simulink library "thermochemical"  (R2017b)
settings: Solver=VariableStepAuto  StartTime=0.0  StopTime=10.0  RelTol=1e-3
values from neighbouring files (symbols this model uses):
  c = conversion_factors()    [blk_clausius_clapeyron.m]    (also in blk_clausius_clapeyron_no_popup.m; blk_cold_room_closed_dry_air.m; blk_reactor_BaCl2_NH3_no_walls.m; blk_reactor_BaCl2_NH3_no_walls_state_space.m)
  cp = metal.cp    [blk_wall_simple.m]    (also in get_metal_properties.m = 390)
  fluid = get_param(blk,'fluid')    [blk_thermodynamic_properties_nonsaturated.m]    (also in blk_thermodynamic_properties_nonsaturated_interpreted.m; blk_thermodynamic_properties_saturated.m; blk_thermodynamic_properties_saturated_interpreted.m; blk_thermodynamic_properties_saturated_mix.m)
  gas = get_material_properties(x.gasName)    [blk_reactor_BaCl2_NH3_cylindrical_no_walls_fun1.m]
  h = get_param(gcb,'ObjectParameters')    [get_param_eval.m]
  rho = metal.rho    [blk_wall_simple.m]    (also in get_metal_properties.m = 8940)
  s = solve(eq,dx,'ReturnConditions',true)    [LMTD_inv.m]    (also in blk_wall_simple.m = get_param_eval(blk,'s'))
  u_gas_at_T_ref = -R * T_ref    [blk_reactor_BaCl2_NH3_no_walls.m]    (also in blk_reactor_BaCl2_NH3_no_walls_state_space.m)
undefined symbols (not defined in the file or in its folder): b_motor, BaCl2, beta, CoolProp, cP_binder, cP_gas, cP_s0, cv, dh_r_0, ENG, heat_exchanger_epsilonNTU_inv_simulink, heat_exchanger_epsilonNTU_simulink, J_motor, K_cin, kappa, Km_motor, La_motor, lookup2D_BreakPoint2, M_binder, N_binder, N_gas_free_volume_init, N_salt, NH3, nh3_v3, nu, P, phase, PID_D_motor, PID_I_motor, PID_P_motor, Ra_motor, Reactor_phase, T, T1, T2, T_init, Tr_init, Tr_ref, U_binder_at_Tr_ref, U_salt_at_X0_Tr_ref, Ur_init, V_void, Valve_regime, Vmax_motor, w_init_motor, X_init
libraries: thermochemical x247, simulink x54, dspsigops x3
(part 3 of 12)

== system thermochemical/Control volumes/Two-phase saturated fluid control volume (with wall, simple) (without algebraic loop) ==
  In2 : Inport
  In5 : Inport  Port=2
  In6 : Inport  Port=3
  In7 : Inport  Port=4
  In1 : Inport  Port=5
  In3 : Inport  Port=6
  In4 : Inport  Port=7
  In8 : Inport  Port=8
  Gain : Gain  Gain=-1
  Subsystem2 : Subsystem
  Two-phase saturated fluid control volume (without walls) (without algebraic loop) : thermochemical/Control volumes/Two-phase saturated fluid control volume (without walls) (without algebraic loop)  N_init=100  T_init=300  fluid=fluid  V=0.01
      settings: SourceProductName=@ Thermochemical
  "Wall, simple, h as inputs" : thermochemical/Walls/Wall, simple, h as inputs  material=Aluminum 1100  cp=905.9  rho=2658  s=1  e_mm=1  mass=2.658  Twall_init=300
      settings: SourceProductName=@ Thermochemical
  Out6 : Outport
  Out4 : Outport  Port=2
  Out11 : Outport  Port=3
  Out7 : Outport  Port=4
  Out5 : Outport  Port=5
  Out12 : Outport  Port=6
  Out13 : Outport  Port=7
  Out8 : Outport  Port=8
  Out1 : Outport  Port=9
  Out10 : Outport  Port=10
  wires:
  In1/1 -> Two-phase saturated fluid control volume (without walls) (without algebraic loop)/5  "dn/dt liq,out (mol/sec) (must be >= 0 !)"
  Gain/1 -> Two-phase saturated fluid control volume (without walls) (without algebraic loop)/1
  In2/1 -> "Wall, simple, h as inputs"/1  "T outer (K)"
  "Wall, simple, h as inputs"/3 -> Out13/1  "q wall → outer (W)"
  In6/1 -> Two-phase saturated fluid control volume (without walls) (without algebraic loop)/3  "dn/dt in (mol/sec) (must be >= 0 !)"
  In5/1 -> Two-phase saturated fluid control volume (without walls) (without algebraic loop)/2  "h in (J/mol)"
  Two-phase saturated fluid control volume (without walls) (without algebraic loop)/3 -> Out5/1, Subsystem2/3(In1)  "liquid volumetric fraction (0..1)"
  Two-phase saturated fluid control volume (without walls) (without algebraic loop)/4 -> Out7/1  "vapor quality (0..1)"
  Two-phase saturated fluid control volume (without walls) (without algebraic loop)/5 -> Out8/1  "h vap (sat) (J/mol)"
  In7/1 -> Two-phase saturated fluid control volume (without walls) (without algebraic loop)/4  "dn/dt vap,out (mol/sec) (must be >= 0 !)"
  Two-phase saturated fluid control volume (without walls) (without algebraic loop)/6 -> Out10/1  "h liq+vap (sat) (J/mol)"
  Two-phase saturated fluid control volume (without walls) (without algebraic loop)/2 -> Out6/1  "P sat (bar)"
  Two-phase saturated fluid control volume (without walls) (without algebraic loop)/1 -> Out4/1, "Wall, simple, h as inputs"/3  "T sat (K)"
  Two-phase saturated fluid control volume (without walls) (without algebraic loop)/7 -> Out1/1  "h liq (sat) (J/mol)"
  "Wall, simple, h as inputs"/1 -> Out11/1  "T wall (K)"
  "Wall, simple, h as inputs"/2 -> Out12/1, Gain/1  "q inner → wall (W)"
  Subsystem2/1(Out1) -> "Wall, simple, h as inputs"/4
  In8/1 -> Subsystem2/2(In3)  "h inner,vap (W/m²/K)"
  In4/1 -> Subsystem2/1(In2)  "h inner,liq (W/m²/K)"
  In3/1 -> "Wall, simple, h as inputs"/2  "h outer (W/m²/K)"

== system thermochemical/Control volumes/Two-phase saturated fluid control volume (with wall, tube with//without fins) ==
  In2 : Inport
  In5 : Inport  Port=2
  In6 : Inport  Port=3
  In7 : Inport  Port=4
  In1 : Inport  Port=5
  In3 : Inport  Port=6
  In4 : Inport  Port=7
  In8 : Inport  Port=8
  Display : Display
  Gain : Gain  Gain=-1
  Subsystem2 : Subsystem
  Two-phase saturated fluid control volume (without walls) : thermochemical/Control volumes/Two-phase saturated fluid control volume (without walls)  N_init=100  T_init=300  fluid=fluid  V=0.01
      settings: SourceProductName=@ Thermochemical
  "Wall, tube with/without fins" : thermochemical/Walls/Wall, tube with//without fins  L_m=1  OD_mm=10  e_mm=1  material_tube=Aluminum 1100  cp_tube=905.9  rho_tube=2658  height_fin_mm=0  thickness_fin_mm=0  pitch_fin_mm=0  material_fin=Aluminum 1100  cp_fin=905.9  rho_fin=2658  lambda_fin=211.8  Tinit=300  mass_tube=0.039664  mass_fin=0  mass_total=0.039664  s_inner=0.028274  s_outer=0.031416
      settings: SourceProductName=@ Thermochemical
  Out6 : Outport
  Out4 : Outport  Port=2
  Out11 : Outport  Port=3
  Out7 : Outport  Port=4
  Out5 : Outport  Port=5
  Out12 : Outport  Port=6
  Out13 : Outport  Port=7
  Out8 : Outport  Port=8
  Out1 : Outport  Port=9
  Out10 : Outport  Port=10
  wires:
  Gain/1 -> Two-phase saturated fluid control volume (without walls)/1
  In2/1 -> "Wall, tube with/without fins"/1  "T outer (K)"
  "Wall, tube with/without fins"/3 -> Out13/1  "q wall → outer (W)"
  Two-phase saturated fluid control volume (without walls)/3 -> Out5/1, Subsystem2/3(In1)  "liquid volumetric fraction (0..1)"
  Two-phase saturated fluid control volume (without walls)/4 -> Out7/1  "vapor quality (0..1)"
  Two-phase saturated fluid control volume (without walls)/5 -> Out8/1  "h vap (sat) (J/mol)"
  Two-phase saturated fluid control volume (without walls)/6 -> Out10/1  "h liq+vap (sat) (J/mol)"
  Two-phase saturated fluid control volume (without walls)/2 -> Out6/1  "P sat (bar)"
  Two-phase saturated fluid control volume (without walls)/1 -> "Wall, tube with/without fins"/3, Out4/1  "T sat (K)"
  Two-phase saturated fluid control volume (without walls)/7 -> Out1/1  "h liq (sat) (J/mol)"
  "Wall, tube with/without fins"/1 -> Out11/1  "T wall (K)"
  "Wall, tube with/without fins"/2 -> Gain/1, Out12/1  "q inner → wall (W)"
  Subsystem2/1(Out1) -> "Wall, tube with/without fins"/4
  "Wall, tube with/without fins"/4 -> Display/1
  In6/1 -> Two-phase saturated fluid control volume (without walls)/3  "dn/dt in (mol/sec) (must be >= 0 !)"
  In7/1 -> Two-phase saturated fluid control volume (without walls)/4  "dn/dt vap,out (mol/sec) (must be >= 0 !)"
  In5/1 -> Two-phase saturated fluid control volume (without walls)/2  "h in (J/mol)"
  In1/1 -> Two-phase saturated fluid control volume (without walls)/5  "dn/dt liq,out (mol/sec) (must be >= 0 !)"
  In8/1 -> Subsystem2/2(In3)  "h inner,vap (W/m²/K)"
  In4/1 -> Subsystem2/1(In2)  "h inner,liq (W/m²/K)"
  In3/1 -> "Wall, tube with/without fins"/2  "h outer (W/m²/K)"

== system thermochemical/Control volumes/Two-phase saturated fluid control volume (with wall, tube with//without fins) (without algebraic loop) ==
  In2 : Inport
  In5 : Inport  Port=2
  In6 : Inport  Port=3
  In7 : Inport  Port=4
  In1 : Inport  Port=5
  In3 : Inport  Port=6
  In4 : Inport  Port=7
  In8 : Inport  Port=8
  Display : Display
  Gain : Gain  Gain=-1
  Subsystem2 : Subsystem
  Two-phase saturated fluid control volume (without walls) (without algebraic loop) : thermochemical/Control volumes/Two-phase saturated fluid control volume (without walls) (without algebraic loop)  N_init=100  T_init=300  fluid=fluid  V=0.01
      settings: SourceProductName=@ Thermochemical
  "Wall, tube with/without fins" : thermochemical/Walls/Wall, tube with//without fins  L_m=1  OD_mm=10  e_mm=1  material_tube=Aluminum 1100  cp_tube=905.9  rho_tube=2658  height_fin_mm=0  thickness_fin_mm=0  pitch_fin_mm=0  material_fin=Aluminum 1100  cp_fin=905.9  rho_fin=2658  lambda_fin=211.8  Tinit=300  mass_tube=0.039664  mass_fin=0  mass_total=0.039664  s_inner=0.028274  s_outer=0.031416
      settings: SourceProductName=@ Thermochemical
  Out6 : Outport
  Out4 : Outport  Port=2
  Out11 : Outport  Port=3
  Out7 : Outport  Port=4
  Out5 : Outport  Port=5
  Out12 : Outport  Port=6
  Out13 : Outport  Port=7
  Out8 : Outport  Port=8
  Out1 : Outport  Port=9
  Out10 : Outport  Port=10
  wires:
  In1/1 -> Two-phase saturated fluid control volume (without walls) (without algebraic loop)/5  "dn/dt liq,out (mol/sec) (must be >= 0 !)"
  In5/1 -> Two-phase saturated fluid control volume (without walls) (without algebraic loop)/2  "h in (J/mol)"
  In7/1 -> Two-phase saturated fluid control volume (without walls) (without algebraic loop)/4  "dn/dt vap,out (mol/sec) (must be >= 0 !)"
  In6/1 -> Two-phase saturated fluid control volume (without walls) (without algebraic loop)/3  "dn/dt in (mol/sec) (must be >= 0 !)"
  "Wall, tube with/without fins"/4 -> Display/1
  Subsystem2/1(Out1) -> "Wall, tube with/without fins"/4
  "Wall, tube with/without fins"/2 -> Out12/1, Gain/1  "q inner → wall (W)"
  "Wall, tube with/without fins"/1 -> Out11/1  "T wall (K)"
  Two-phase saturated fluid control volume (without walls) (without algebraic loop)/7 -> Out1/1  "h liq (sat) (J/mol)"
  Two-phase saturated fluid control volume (without walls) (without algebraic loop)/1 -> Out4/1, "Wall, tube with/without fins"/3  "T sat (K)"
  Two-phase saturated fluid control volume (without walls) (without algebraic loop)/2 -> Out6/1  "P sat (bar)"
  Two-phase saturated fluid control volume (without walls) (without algebraic loop)/6 -> Out10/1  "h liq+vap (sat) (J/mol)"
  Two-phase saturated fluid control volume (without walls) (without algebraic loop)/5 -> Out8/1  "h vap (sat) (J/mol)"
  Two-phase saturated fluid control volume (without walls) (without algebraic loop)/4 -> Out7/1  "vapor quality (0..1)"
  Two-phase saturated fluid control volume (without walls) (without algebraic loop)/3 -> Subsystem2/3(In1), Out5/1  "liquid volumetric fraction (0..1)"
  "Wall, tube with/without fins"/3 -> Out13/1  "q wall → outer (W)"
  In2/1 -> "Wall, tube with/without fins"/1  "T outer (K)"
  Gain/1 -> Two-phase saturated fluid control volume (without walls) (without algebraic loop)/1
  In8/1 -> Subsystem2/2(In3)  "h inner,vap (W/m²/K)"
  In4/1 -> Subsystem2/1(In2)  "h inner,liq (W/m²/K)"
  In3/1 -> "Wall, tube with/without fins"/2  "h outer (W/m²/K)"

== system thermochemical/Control volumes/Two-phase saturated fluid control volume (without walls) ==
  In6 : Inport
  In7 : Inport  Port=2
  In8 : Inport  Port=3
  In9 : Inport  Port=4
  In11 : Inport  Port=5
  1 : Constant  Value=N_init
  Heat exchanger's temperature and liquid level : Subsystem
  Integrator1 : Integrator  InitialConditionSource=external  InitialCondition=N_init
  Internal energy differential equation : Subsystem
  Sum1 : Sum  Inputs=+--
  Thermodynamic property (saturated)1 : thermochemical/Thermodynamic fluid properties/Thermodynamic  property (saturated)  sel=h(T) vap. (J/mol)  fluid=fluid  lookup1D_BreakPoint1=fluid.sat.T  lookup1D_Data=fluid.sat.vap.h_molar
      settings: SourceProductName=@ Thermochemical
  Thermodynamic property (saturated)2 : thermochemical/Thermodynamic fluid properties/Thermodynamic  property (saturated)  sel=P(T) (bar)  fluid=fluid  lookup1D_BreakPoint1=fluid.sat.T  lookup1D_Data=fluid.sat.Psat
      settings: SourceProductName=@ Thermochemical
  Thermodynamic property (saturated)3 : thermochemical/Thermodynamic fluid properties/Thermodynamic  property (saturated)  sel=h(T) liq. (J/mol)  fluid=fluid  lookup1D_BreakPoint1=fluid.sat.T  lookup1D_Data=fluid.sat.liq.h_molar
      settings: SourceProductName=@ Thermochemical
  Thermodynamic property (saturated vapor-liquid mix) : thermochemical/Thermodynamic fluid properties/Thermodynamic property  (saturated vapor-liquid mix)  sel=h(T) (J/mol)  fluid=fluid  lookup1D_BreakPoint=0  lookup1D_Data1=fluid.sat.liq.h_molar  lookup1D_Data2=fluid.sat.vap.h_molar
      settings: SourceProductName=@ Thermochemical
  Out2 : Outport
  Out3 : Outport  Port=2
  Out1 : Outport  Port=3
  Out4 : Outport  Port=4
  Out5 : Outport  Port=5
  Out7 : Outport  Port=6
  Out6 : Outport  Port=7
  wires:
  Sum1/1 -> Integrator1/1
  Heat exchanger's temperature and liquid level/3(Out2) -> Out1/1  "liquid volumetric fraction (0..1)"
  Heat exchanger's temperature and liquid level/1(Out1) -> Thermodynamic property (saturated)3/1, Thermodynamic property (saturated)1/1, Thermodynamic property (saturated)2/1, Out2/1, Thermodynamic property (saturated vapor-liquid mix)/1  "T sat (K)"
  Thermodynamic property (saturated)2/1 -> Out3/1  "P sat (bar)"
  Heat exchanger's temperature and liquid level/2(Out3) -> Thermodynamic property (saturated vapor-liquid mix)/2, Out4/1  "vapor quality (0..1)"
  Integrator1/1 -> Heat exchanger's temperature and liquid level/1(In2)  "N hx"
  Internal energy differential equation/1(Out1) -> Heat exchanger's temperature and liquid level/2(In1)
  Thermodynamic property (saturated)1/1 -> Internal energy differential equation/4(In5), Out5/1  "h vap (J/mol)"
  Thermodynamic property (saturated vapor-liquid mix)/1 -> Out7/1  "h liq+vap (J/mol)"
  Thermodynamic property (saturated)3/1 -> Out6/1, Internal energy differential equation/6(In7)  "h liq (J/mol)"
  In9/1 -> Sum1/2, Internal energy differential equation/5(In4)  "dn/dt vap,out (mol/sec)"
  In6/1 -> Internal energy differential equation/1(In1)  "q wall → exchanger (W)"
  In8/1 -> Sum1/1, Internal energy differential equation/3(In3)  "dn/dt in (mol/sec)"
  In11/1 -> Sum1/3, Internal energy differential equation/7(In6)  "dn/dt liq,out (mol/sec)"
  In7/1 -> Internal energy differential equation/2(In2)  "h in (J/mol)"
  1/1 -> Integrator1/2

== system thermochemical/Control volumes/Two-phase saturated fluid control volume (without walls) (without algebraic loop) ==
  In6 : Inport
  In7 : Inport  Port=2
  In8 : Inport  Port=3
  In9 : Inport  Port=4
  In11 : Inport  Port=5
  Demux : Demux  Outputs=7
  Initial condition vector : Constant  Value=[T_init; V/N_init]
  Integrator2 : Integrator  InitialConditionSource=external
  Mux : Mux  Inputs=5
  Reactor output function : Subsystem
  Two-phase control volume state-space functions : Subsystem
  Out2 : Outport
  Out3 : Outport  Port=2
  Out1 : Outport  Port=3
  Out4 : Outport  Port=4
  Out5 : Outport  Port=5
  Out7 : Outport  Port=6
  Out6 : Outport  Port=7
  wires:
  Integrator2/1 -> Two-phase control volume state-space functions/1(In1), Reactor output function/1(In1)  "X"
  Initial condition vector/1 -> Integrator2/2
  Two-phase control volume state-space functions/1(Out2) -> Integrator2/1
  Mux/1 -> Two-phase control volume state-space functions/2(In2)
  Reactor output function/1(Out1) -> Demux/1  "Y"
  Demux/7 -> Out6/1  "h liq (J/mol)"
  Demux/2 -> Out3/1  "P (bar)"
  Demux/6 -> Out7/1  "h liq+vap (J/mol)"
  Demux/5 -> Out5/1  "h vap (J/mol)"
  Demux/4 -> Out4/1  "vapor quality (0..1)"
  Demux/1 -> Out2/1  "T (K)"
  Demux/3 -> Out1/1  "liquid volumetric fraction (0..1)"
  In6/1 -> Mux/1  "q wall → exchanger (W)"
  In11/1 -> Mux/5  "dn/dt liq,out (mol/sec)"
  In8/1 -> Mux/3  "dn/dt in (mol/sec)"
  In7/1 -> Mux/2  "h in (J/mol)"
  In9/1 -> Mux/4  "dn/dt vap,out (mol/sec)"

== system thermochemical/Control volumes/Two-phase saturated fluid control volume energy equation ==
  In2 : Inport
  In3 : Inport  Port=2
  In1 : Inport  Port=3
  Product4 : Product
  Thermodynamic property (saturated vapor-liquid mix) : thermochemical/Thermodynamic fluid properties/Thermodynamic property  (saturated vapor-liquid mix)  sel=u(T) (J/mol)  fluid=fluid  lookup1D_BreakPoint=0  lookup1D_Data1=fluid.sat.liq.u_molar  lookup1D_Data2=fluid.sat.vap.u_molar
      settings: SourceProductName=@ Thermochemical
  Vapor quality & Liquid volumetric fraction : thermochemical/Thermodynamic fluid properties/Vapor quality & Liquid  volumetric fraction  fluid=fluid
      settings: SourceProductName=@ Thermochemical
  Out1 : Outport
  Out2 : Outport  Port=2
  Out3 : Outport  Port=3
  wires:
  In1/1 -> Thermodynamic property (saturated vapor-liquid mix)/1, Vapor quality & Liquid volumetric fraction/1  "T (K)"
  In2/1 -> Vapor quality & Liquid volumetric fraction/2, Product4/1  "N (mol)"
  Vapor quality & Liquid volumetric fraction/2 -> Out2/1  "liquid volumetric fraction (0..1)"
  In3/1 -> Vapor quality & Liquid volumetric fraction/3  "V (m3)"
  Vapor quality & Liquid volumetric fraction/1 -> Out3/1, Thermodynamic property (saturated vapor-liquid mix)/2  "vapor quality (0..1)"
  Thermodynamic property (saturated vapor-liquid mix)/1 -> Product4/2
  Product4/1 -> Out1/1  "U (J)"

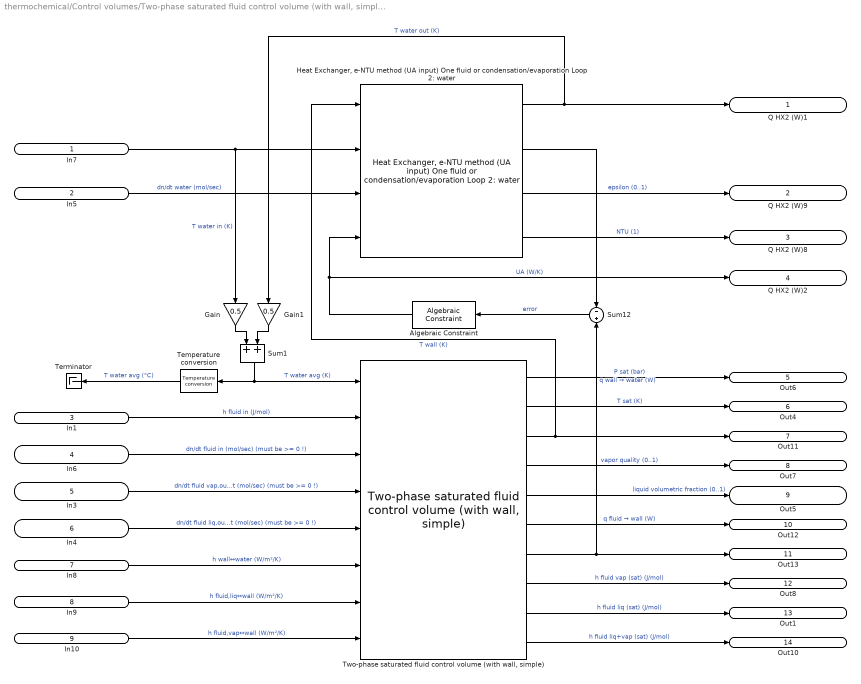
== system thermochemical/Control volumes/Two-phase saturated fluid control volume (with wall, simple) + heat exchanger (condensation//evaporation), with water loop ==
  In7 : Inport
  In5 : Inport  Port=2
  In1 : Inport  Port=3
  In6 : Inport  Port=4
  In3 : Inport  Port=5
  In4 : Inport  Port=6
  In8 : Inport  Port=7
  In9 : Inport  Port=8
  In10 : Inport  Port=9
  Algebraic Constraint : AlgebraicConstraint  Solver=Trust region  InitialGuess=1
  Gain : Gain  Gain=0.5
  Gain1 : Gain  Gain=0.5
  "Heat Exchanger, e-NTU method (UA input) One fluid or condensation/evaporation Loop 2: water" : thermochemical/Heat exchangers/Heat Exchanger, e-NTU method (UA input) One fluid or condensation//evaporation Loop 2: water  cp_water_J_K_mol=75.3260
      settings: SourceProductName=@ Thermochemical
  Sum1 : Sum
  Sum12 : Sum  Inputs=-+
  Temperature conversion : thermochemical/Conversions/Temperature conversion  sel=K --> °C
      settings: SourceProductName=@ Thermochemical
  Terminator : Terminator
  "Two-phase saturated fluid control volume (with wall, simple)" : thermochemical/Control volumes/Two-phase saturated fluid control volume (with wall, simple)
      settings: SourceProductName=@ Thermochemical
  Q HX2 (W)1 : Outport
  Q HX2 (W)9 : Outport  Port=2
  Q HX2 (W)8 : Outport  Port=3
  Q HX2 (W)2 : Outport  Port=4
  Out6 : Outport  Port=5
  Out4 : Outport  Port=6
  Out11 : Outport  Port=7
  Out7 : Outport  Port=8
  Out5 : Outport  Port=9
  Out12 : Outport  Port=10
  Out13 : Outport  Port=11
  Out8 : Outport  Port=12
  Out1 : Outport  Port=13
  Out10 : Outport  Port=14
  wires:
  Sum12/1 -> Algebraic Constraint/1  "error"
  "Two-phase saturated fluid control volume (with wall, simple)"/8 -> Out8/1  "h fluid vap (sat) (J/mol)"
  "Two-phase saturated fluid control volume (with wall, simple)"/7 -> Out13/1, Sum12/2  "q wall → water (W)"
  "Two-phase saturated fluid control volume (with wall, simple)"/4 -> Out7/1  "vapor quality (0..1)"
  "Two-phase saturated fluid control volume (with wall, simple)"/5 -> Out5/1  "liquid volumetric fraction (0..1)"
  "Two-phase saturated fluid control volume (with wall, simple)"/2 -> Out4/1  "T sat (K)"
  "Two-phase saturated fluid control volume (with wall, simple)"/9 -> Out1/1  "h fluid liq (sat) (J/mol)"
  "Two-phase saturated fluid control volume (with wall, simple)"/1 -> Out6/1  "P sat (bar)"
  "Two-phase saturated fluid control volume (with wall, simple)"/3 -> Out11/1, "Heat Exchanger, e-NTU method (UA input) One fluid or condensation/evaporation Loop 2: water"/1  "T wall (K)"
  "Two-phase saturated fluid control volume (with wall, simple)"/10 -> Out10/1  "h fluid liq+vap (sat) (J/mol)"
  "Two-phase saturated fluid control volume (with wall, simple)"/6 -> Out12/1  "q fluid → wall (W)"
  "Heat Exchanger, e-NTU method (UA input) One fluid or condensation/evaporation Loop 2: water"/2 -> Sum12/1
  "Heat Exchanger, e-NTU method (UA input) One fluid or condensation/evaporation Loop 2: water"/1 -> Gain1/1, Q HX2 (W)1/1  "T water out (K)"
  "Heat Exchanger, e-NTU method (UA input) One fluid or condensation/evaporation Loop 2: water"/4 -> Q HX2 (W)8/1  "NTU (1)"
  "Heat Exchanger, e-NTU method (UA input) One fluid or condensation/evaporation Loop 2: water"/3 -> Q HX2 (W)9/1  "epsilon (0..1)"
  Algebraic Constraint/1 -> "Heat Exchanger, e-NTU method (UA input) One fluid or condensation/evaporation Loop 2: water"/4, Q HX2 (W)2/1  "UA (W/K)"
  In10/1 -> "Two-phase saturated fluid control volume (with wall, simple)"/8  "h fluid,vap↔wall (W/m²/K)"
  In8/1 -> "Two-phase saturated fluid control volume (with wall, simple)"/6  "h wall↔water (W/m²/K)"
  In4/1 -> "Two-phase saturated fluid control volume (with wall, simple)"/5  "dn/dt fluid liq,out (mol/sec) (must be >= 0 !)"
  In9/1 -> "Two-phase saturated fluid control volume (with wall, simple)"/7  "h fluid,liq↔wall (W/m²/K)"
  In3/1 -> "Two-phase saturated fluid control volume (with wall, simple)"/4  "dn/dt fluid vap,out (mol/sec) (must be >= 0 !)"
  In1/1 -> "Two-phase saturated fluid control volume (with wall, simple)"/2  "h fluid in (J/mol)"
  In6/1 -> "Two-phase saturated fluid control volume (with wall, simple)"/3  "dn/dt fluid in (mol/sec) (must be >= 0 !)"
  In5/1 -> "Heat Exchanger, e-NTU method (UA input) One fluid or condensation/evaporation Loop 2: water"/3  "dn/dt water (mol/sec)"
  In7/1 -> Gain/1, "Heat Exchanger, e-NTU method (UA input) One fluid or condensation/evaporation Loop 2: water"/2  "T water in (K)"
  Sum1/1 -> Temperature conversion/1, "Two-phase saturated fluid control volume (with wall, simple)"/1  "T water avg (K)"
  Gain/1 -> Sum1/1
  Gain1/1 -> Sum1/2
  Temperature conversion/1 -> Terminator/1  "T water avg (°C)"

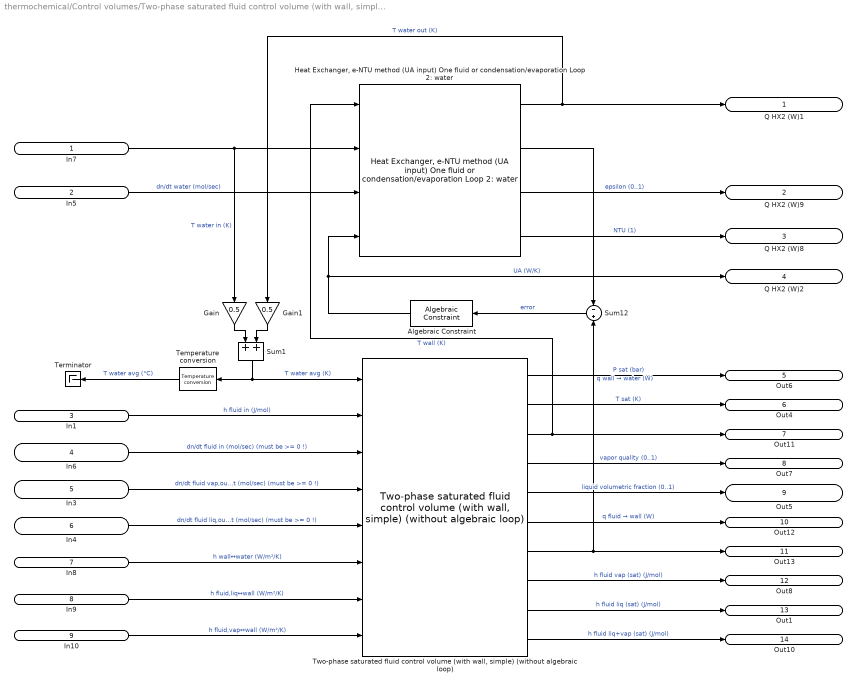
== system thermochemical/Control volumes/Two-phase saturated fluid control volume (with wall, simple) + heat exchanger (condensation//evaporation), with water loop (without algebraic loop) ==
  In7 : Inport
  In5 : Inport  Port=2
  In1 : Inport  Port=3
  In6 : Inport  Port=4
  In3 : Inport  Port=5
  In4 : Inport  Port=6
  In8 : Inport  Port=7
  In9 : Inport  Port=8
  In10 : Inport  Port=9
  Algebraic Constraint : AlgebraicConstraint  Solver=Trust region  InitialGuess=1
  Gain : Gain  Gain=0.5
  Gain1 : Gain  Gain=0.5
  "Heat Exchanger, e-NTU method (UA input) One fluid or condensation/evaporation Loop 2: water" : thermochemical/Heat exchangers/Heat Exchanger, e-NTU method (UA input) One fluid or condensation//evaporation Loop 2: water  cp_water_J_K_mol=75.3260
      settings: SourceProductName=@ Thermochemical
  Sum1 : Sum
  Sum12 : Sum  Inputs=-+
  Temperature conversion : thermochemical/Conversions/Temperature conversion  sel=K --> °C
      settings: SourceProductName=@ Thermochemical
  Terminator : Terminator
  "Two-phase saturated fluid control volume (with wall, simple) (without algebraic loop)" : thermochemical/Control volumes/Two-phase saturated fluid control volume (with wall, simple) (without algebraic loop)
      settings: SourceProductName=@ Thermochemical
  Q HX2 (W)1 : Outport
  Q HX2 (W)9 : Outport  Port=2
  Q HX2 (W)8 : Outport  Port=3
  Q HX2 (W)2 : Outport  Port=4
  Out6 : Outport  Port=5
  Out4 : Outport  Port=6
  Out11 : Outport  Port=7
  Out7 : Outport  Port=8
  Out5 : Outport  Port=9
  Out12 : Outport  Port=10
  Out13 : Outport  Port=11
  Out8 : Outport  Port=12
  Out1 : Outport  Port=13
  Out10 : Outport  Port=14
  wires:
  Gain1/1 -> Sum1/2
  Gain/1 -> Sum1/1
  In7/1 -> "Heat Exchanger, e-NTU method (UA input) One fluid or condensation/evaporation Loop 2: water"/2, Gain/1  "T water in (K)"
  In5/1 -> "Heat Exchanger, e-NTU method (UA input) One fluid or condensation/evaporation Loop 2: water"/3  "dn/dt water (mol/sec)"
  In6/1 -> "Two-phase saturated fluid control volume (with wall, simple) (without algebraic loop)"/3  "dn/dt fluid in (mol/sec) (must be >= 0 !)"
  In1/1 -> "Two-phase saturated fluid control volume (with wall, simple) (without algebraic loop)"/2  "h fluid in (J/mol)"
  In3/1 -> "Two-phase saturated fluid control volume (with wall, simple) (without algebraic loop)"/4  "dn/dt fluid vap,out (mol/sec) (must be >= 0 !)"
  In9/1 -> "Two-phase saturated fluid control volume (with wall, simple) (without algebraic loop)"/7  "h fluid,liq↔wall (W/m²/K)"
  In4/1 -> "Two-phase saturated fluid control volume (with wall, simple) (without algebraic loop)"/5  "dn/dt fluid liq,out (mol/sec) (must be >= 0 !)"
  In8/1 -> "Two-phase saturated fluid control volume (with wall, simple) (without algebraic loop)"/6  "h wall↔water (W/m²/K)"
  In10/1 -> "Two-phase saturated fluid control volume (with wall, simple) (without algebraic loop)"/8  "h fluid,vap↔wall (W/m²/K)"
  Algebraic Constraint/1 -> Q HX2 (W)2/1, "Heat Exchanger, e-NTU method (UA input) One fluid or condensation/evaporation Loop 2: water"/4  "UA (W/K)"
  "Heat Exchanger, e-NTU method (UA input) One fluid or condensation/evaporation Loop 2: water"/3 -> Q HX2 (W)9/1  "epsilon (0..1)"
  "Heat Exchanger, e-NTU method (UA input) One fluid or condensation/evaporation Loop 2: water"/4 -> Q HX2 (W)8/1  "NTU (1)"
  "Heat Exchanger, e-NTU method (UA input) One fluid or condensation/evaporation Loop 2: water"/1 -> Q HX2 (W)1/1, Gain1/1  "T water out (K)"
  "Heat Exchanger, e-NTU method (UA input) One fluid or condensation/evaporation Loop 2: water"/2 -> Sum12/1
  "Two-phase saturated fluid control volume (with wall, simple) (without algebraic loop)"/6 -> Out12/1  "q fluid → wall (W)"
  "Two-phase saturated fluid control volume (with wall, simple) (without algebraic loop)"/10 -> Out10/1  "h fluid liq+vap (sat) (J/mol)"
  "Two-phase saturated fluid control volume (with wall, simple) (without algebraic loop)"/3 -> "Heat Exchanger, e-NTU method (UA input) One fluid or condensation/evaporation Loop 2: water"/1, Out11/1  "T wall (K)"
  "Two-phase saturated fluid control volume (with wall, simple) (without algebraic loop)"/1 -> Out6/1  "P sat (bar)"
  "Two-phase saturated fluid control volume (with wall, simple) (without algebraic loop)"/9 -> Out1/1  "h fluid liq (sat) (J/mol)"
  "Two-phase saturated fluid control volume (with wall, simple) (without algebraic loop)"/2 -> Out4/1  "T sat (K)"
  "Two-phase saturated fluid control volume (with wall, simple) (without algebraic loop)"/5 -> Out5/1  "liquid volumetric fraction (0..1)"
  "Two-phase saturated fluid control volume (with wall, simple) (without algebraic loop)"/4 -> Out7/1  "vapor quality (0..1)"
  "Two-phase saturated fluid control volume (with wall, simple) (without algebraic loop)"/7 -> Sum12/2, Out13/1  "q wall → water (W)"
  "Two-phase saturated fluid control volume (with wall, simple) (without algebraic loop)"/8 -> Out8/1  "h fluid vap (sat) (J/mol)"
  Sum12/1 -> Algebraic Constraint/1  "error"
  Temperature conversion/1 -> Terminator/1  "T water avg (°C)"
  Sum1/1 -> Temperature conversion/1, "Two-phase saturated fluid control volume (with wall, simple) (without algebraic loop)"/1  "T water avg (K)"

== system thermochemical/Conversions/Pressure conversion ==
  In1 : Inport
  Gain : Gain  Gain=1e-05
  Out1 : Outport
  wires:
  In1/1 -> Gain/1  "(Pa)"
  Gain/1 -> Out1/1  "(bar)"

== system thermochemical/Conversions/Rotational speed conversion ==
  In1 : Inport
  Gain : Gain  Gain=0.10472
  Out1 : Outport
  wires:
  Gain/1 -> Out1/1  "(rad/sec)"
  In1/1 -> Gain/1  "(rpm)"

== system thermochemical/Conversions/Temperature conversion ==
  In1 : Inport
  Constant : Constant  Value=9
  Multiport Switch : MultiPortSwitch  Inputs=12
  Subsystem : Subsystem
  Subsystem1 : Subsystem
  Subsystem10 : thermochemical/Conversions/Temperature conversion/Subsystem3
      settings: SourceProductName=@ Thermochemical
  Subsystem11 : thermochemical/Conversions/Temperature conversion/Subsystem2
      settings: SourceProductName=@ Thermochemical
  Subsystem12 : thermochemical/Conversions/Temperature conversion/Subsystem5
      settings: SourceProductName=@ Thermochemical
  Subsystem13 : thermochemical/Conversions/Temperature conversion/Subsystem4
      settings: SourceProductName=@ Thermochemical
  Subsystem14 : thermochemical/Conversions/Temperature conversion/Subsystem4
      settings: SourceProductName=@ Thermochemical
  Subsystem15 : thermochemical/Conversions/Temperature conversion/Subsystem2
      settings: SourceProductName=@ Thermochemical
  Subsystem16 : thermochemical/Conversions/Temperature conversion/Subsystem
      settings: SourceProductName=@ Thermochemical
  Subsystem17 : thermochemical/Conversions/Temperature conversion/Subsystem5
      settings: SourceProductName=@ Thermochemical
  Subsystem18 : thermochemical/Conversions/Temperature conversion/Subsystem3
      settings: SourceProductName=@ Thermochemical
  Subsystem19 : thermochemical/Conversions/Temperature conversion/Subsystem1
      settings: SourceProductName=@ Thermochemical
  Subsystem2 : Subsystem
  Subsystem3 : Subsystem
  Subsystem4 : Subsystem
  Subsystem5 : Subsystem
  Subsystem6 : thermochemical/Conversions/Temperature conversion/Subsystem2
      settings: SourceProductName=@ Thermochemical
  Subsystem7 : thermochemical/Conversions/Temperature conversion/Subsystem
      settings: SourceProductName=@ Thermochemical
  Subsystem8 : thermochemical/Conversions/Temperature conversion/Subsystem3
      settings: SourceProductName=@ Thermochemical
  Subsystem9 : thermochemical/Conversions/Temperature conversion/Subsystem1
      settings: SourceProductName=@ Thermochemical
  Out1 : Outport
  wires:
  Multiport Switch/1 -> Out1/1  "(°F)"
  Constant/1 -> Multiport Switch/1
  In1/1 -> Subsystem8/1, Subsystem7/1, Subsystem3/1((K)), Subsystem2/1((K)), Subsystem1/1((K)), Subsystem/1((K)), Subsystem11/1, Subsystem12/1, Subsystem13/1, Subsystem17/1, Subsystem16/1, Subsystem5/1((K))  "(°R)"
  Subsystem/1((°C)) -> Multiport Switch/2
  Subsystem1/1((°C)) -> Multiport Switch/3
  Subsystem2/1((°C)) -> Multiport Switch/4
  Subsystem3/1((°C)) -> Multiport Switch/5
  Subsystem7/1 -> Subsystem6/1
  Subsystem6/1 -> Multiport Switch/6
  Subsystem8/1 -> Subsystem9/1
  Subsystem9/1 -> Multiport Switch/7
  Subsystem5/1((°C)) -> Subsystem10/1
  Subsystem10/1 -> Multiport Switch/8
  Subsystem11/1 -> Subsystem4/1((K))
  Subsystem4/1((°C)) -> Multiport Switch/9
  Subsystem12/1 -> Multiport Switch/10
  Subsystem13/1 -> Multiport Switch/11
  Subsystem14/1 -> Multiport Switch/12
  Subsystem15/1 -> Subsystem14/1
  Subsystem16/1 -> Subsystem15/1
  Subsystem17/1 -> Subsystem18/1
  Subsystem18/1 -> Subsystem19/1
  Subsystem19/1 -> Multiport Switch/13

== system thermochemical/Conversions/Volume flow rate conversion ==
  In1 : Inport
  Gain : Gain  Gain=0.58858
  Out1 : Outport
  wires:
  Gain/1 -> Out1/1  "(CFM)"
  In1/1 -> Gain/1  "(m3/h)"

== system thermochemical/Heat exchangers/Heat Exchanger, e-NTU method (UA input) (it uses CoolProp library) ==
  dN/dt comp (mol/sec) : Inport
  dN/dt comp (mol/sec)1 : Inport  Port=2
  dN/dt comp (mol/sec)2 : Inport  Port=3
  dN/dt comp (mol/sec)3 : Inport  Port=4
  dN/dt comp (mol/sec)4 : Inport  Port=5
  dN/dt comp (mol/sec)5 : Inport  Port=6
  dN/dt comp (mol/sec)6 : Inport  Port=7
  Demux : Demux  Outputs=7
  Display10 : Display
  Mux2 : Mux  Inputs=7
  heat_exchanger : MATLABFcn  MATLABFcn=heat_exchanger_epsilonNTU_simulink(u(1),u(2),u(3),'Water',u(4),u(5),u(6),'Water',u(7),'Counter-flow')  OutputDimensions=7  OutputSignalType=real
  Q HX2 (W)1 : Outport
  Q HX2 (W)2 : Outport  Port=2
  Q HX2 (W)3 : Outport  Port=3
  Q HX2 (W)4 : Outport  Port=4
  Q HX2 (W)6 : Outport  Port=5
  Q HX2 (W)5 : Outport  Port=6
  Q HX2 (W)7 : Outport  Port=7
  wires:
  Demux/4 -> Q HX2 (W)4/1  "epsilon (0..1)"
  Demux/2 -> Q HX2 (W)2/1  "T2,out (K)"
  Mux2/1 -> heat_exchanger/1
  Demux/3 -> Q HX2 (W)3/1  "q1→2 (W)"
  Demux/7 -> Q HX2 (W)5/1, Display10/1  "minimization residue"
  dN/dt comp (mol/sec)5/1 -> Mux2/6  "dN/dt 2 (mol/sec)"
  dN/dt comp (mol/sec)6/1 -> Mux2/7  "U*A (W/K)"
  dN/dt comp (mol/sec)4/1 -> Mux2/5  "P2 (bar)"
  dN/dt comp (mol/sec)3/1 -> Mux2/4  "T2,in (K)"
  dN/dt comp (mol/sec)/1 -> Mux2/1  "T1,in (K)"
  dN/dt comp (mol/sec)1/1 -> Mux2/2  "P1 (bar)"
  Demux/1 -> Q HX2 (W)1/1  "T1,out (K)"
  heat_exchanger/1 -> Demux/1
  dN/dt comp (mol/sec)2/1 -> Mux2/3  "dN/dt 1 (mol/sec)"
  Demux/5 -> Q HX2 (W)6/1  "NTU (0..Inf)"
  Demux/6 -> Q HX2 (W)7/1  "Cr (0..1)"

== system thermochemical/Heat exchangers/Heat Exchanger, e-NTU method (UA input) Loop 2: water ==
  In1 : Inport
  In3 : Inport  Port=2
  In4 : Inport  Port=3
  In7 : Inport  Port=4
  In5 : Inport  Port=5
  In6 : Inport  Port=6
  Algebraic Constraint : AlgebraicConstraint  InitialGuess=300
  Display : Display
  Product : Product  Inputs=*/
  Product1 : Product  Inputs=*/
  Subsystem : Subsystem
  Sum1 : Sum  Inputs=+-|
  Sum2 : Sum  Inputs=++|
  Sum3 : Sum  Inputs=|-+
  Q HX2 (W)7 : Outport
  Q HX2 (W)1 : Outport  Port=2
  Q HX2 (W)4 : Outport  Port=3
  Q HX2 (W)9 : Outport  Port=4
  Q HX2 (W)8 : Outport  Port=5
  Q HX2 (W)2 : Outport  Port=6
  Q HX2 (W)11 : Outport  Port=7
  wires:
  Algebraic Constraint/1 -> Subsystem/2(In2), Sum3/2  "T1 out ** (K)"
  Sum3/1 -> Algebraic Constraint/1, Q HX2 (W)2/1  "minimization residue"
  Product/1 -> Sum1/2  "Q * C1"
  Sum2/1 -> Q HX2 (W)1/1  "T water out (K)"
  Product1/1 -> Sum2/2  "Q * C2"
  Subsystem/7(Q HX2 (W)6) -> Product1/2
  In7/1 -> Sum2/1, Subsystem/7(In7)  "T water in (K)"
  Subsystem/5(Q HX2 (W)4) -> Product1/1, Product/1, Q HX2 (W)4/1  "q1→water (W)"
  Subsystem/3(Q HX2 (W)10) -> Display/1  "q1→water max (W)"
  In4/1 -> Subsystem/4(In4)  "dn/dt 1 (mol/sec)"
  Subsystem/4(Q HX2 (W)11) -> Q HX2 (W)11/1  "Cr (0..1)"
  In3/1 -> Subsystem/3(In3)  "P1 in = P1 out (bar)"
  In5/1 -> Subsystem/5(In5)  "dn/dt water (mol/sec)"
  Subsystem/2(Q HX2 (W)8) -> Q HX2 (W)9/1  "epsilon (0..1)"
  Subsystem/1(Q HX2 (W)9) -> Q HX2 (W)8/1  "NTU (1)"
  In6/1 -> Subsystem/6(In6)  "UA (W/K)"
  Sum1/1 -> Q HX2 (W)7/1, Sum3/1  "T1 out (K)"
  In1/1 -> Sum1/1, Subsystem/1(In1)  "T1 in (K)"
  Subsystem/6(Q HX2 (W)3) -> Product/2

== system thermochemical/Heat exchangers/Heat Exchanger, e-NTU method (UA input) One fluid or condensation//evaporation Loop 2: water ==
  In1 : Inport
  In7 : Inport  Port=2
  In5 : Inport  Port=3
  In6 : Inport  Port=4
  Display : Display
  NTU : Subsystem
  Product1 : Product
  Product2 : Product
  Product3 : Product
  Product4 : Product  Inputs=/*
  Product5 : Product  Inputs=/*
  Sum : Sum  Inputs=+-
  Sum1 : Sum  Inputs=|++
  cp water (J/K·mol) : Constant  Value=cp_water_J_K_mol
  Q HX2 (W)1 : Outport
  Q HX2 (W)4 : Outport  Port=2
  Q HX2 (W)9 : Outport  Port=3
  Q HX2 (W)8 : Outport  Port=4
  wires:
  Product4/1 -> Sum1/2
  NTU/1(Q HX2 (W)8) -> Q HX2 (W)9/1, Product2/2  "epsilon (0..1)"
  Product1/1 -> Product2/1, Display/1  "q1→2 max (W)"
  Sum/1 -> Product1/1
  Product3/1 -> Product1/2, Product4/1, Product5/1  "Cmin (W/K)"
  cp water (J/K·mol)/1 -> Product3/1  "cp2 avg (J/K·mol)"
  Sum1/1 -> Q HX2 (W)1/1  "T water out (K)"
  In1/1 -> Sum/1  "T isotherm (K)"
  In6/1 -> Product5/2  "UA (W/K)"
  In5/1 -> Product3/2  "dn/dt water (mol/sec)"
  Product2/1 -> Q HX2 (W)4/1, Product4/2  "q1→water (W)"
  In7/1 -> Sum/2, Sum1/1  "T water in (K)"
  Product5/1 -> NTU/1(In6), Q HX2 (W)8/1  "NTU (1)"

== system thermochemical/Heat exchangers/Heat Exchanger, e-NTU method (epsilon input) (it uses CoolProp library) ==
  dN/dt comp (mol/sec) : Inport
  dN/dt comp (mol/sec)1 : Inport  Port=2
  dN/dt comp (mol/sec)2 : Inport  Port=3
  dN/dt comp (mol/sec)3 : Inport  Port=4
  dN/dt comp (mol/sec)4 : Inport  Port=5
  dN/dt comp (mol/sec)5 : Inport  Port=6
  dN/dt comp (mol/sec)6 : Inport  Port=7
  Demux : Demux  Outputs=7
  Display10 : Display
  Mux2 : Mux  Inputs=7
  heat_exchanger : MATLABFcn  MATLABFcn=heat_exchanger_epsilonNTU_inv_simulink(u(1),u(2),u(3),'Water',u(4),u(5),u(6),'Water',u(7),'Counter-flow')  OutputDimensions=7  OutputSignalType=real
  Q HX2 (W)1 : Outport
  Q HX2 (W)2 : Outport  Port=2
  Q HX2 (W)3 : Outport  Port=3
  Q HX2 (W)4 : Outport  Port=4
  Q HX2 (W)6 : Outport  Port=5
  Q HX2 (W)5 : Outport  Port=6
  Q HX2 (W)7 : Outport  Port=7
  wires:
  dN/dt comp (mol/sec)2/1 -> Mux2/3  "dn/dt 1 (mol/sec)"
  heat_exchanger/1 -> Demux/1
  Demux/1 -> Q HX2 (W)1/1  "T1,out (K)"
  dN/dt comp (mol/sec)1/1 -> Mux2/2  "P1 (bar)"
  dN/dt comp (mol/sec)/1 -> Mux2/1  "T1,in (K)"
  dN/dt comp (mol/sec)3/1 -> Mux2/4  "T2,in (K)"
  dN/dt comp (mol/sec)4/1 -> Mux2/5  "P2 (bar)"
  dN/dt comp (mol/sec)6/1 -> Mux2/7  "epsilon (0..1)"
  dN/dt comp (mol/sec)5/1 -> Mux2/6  "dn/dt 2 (mol/sec)"
  Demux/7 -> Display10/1, Q HX2 (W)5/1  "minimization residue"
  Demux/3 -> Q HX2 (W)3/1  "q1→2 (W)"
  Mux2/1 -> heat_exchanger/1
  Demux/2 -> Q HX2 (W)2/1  "T2,out (K)"
  Demux/4 -> Q HX2 (W)4/1  "U*A (W/K)"
  Demux/5 -> Q HX2 (W)6/1  "NTU (0..Inf)"
  Demux/6 -> Q HX2 (W)7/1  "Cr (0..1)"

== system thermochemical/Heat exchangers/Heat Exchanger, e-NTU method (epsilon input) Loop 2: water ==
  In1 : Inport
  In3 : Inport  Port=2
  In4 : Inport  Port=3
  In7 : Inport  Port=4
  In5 : Inport  Port=5
  In6 : Inport  Port=6
  Algebraic Constraint : AlgebraicConstraint  InitialGuess=300
  Constant : Constant  Value=0
  Display : Display
  Product : Product  Inputs=*/
  Product1 : Product  Inputs=*/
  Subsystem : Subsystem
  Sum1 : Sum  Inputs=+-|
  Sum2 : Sum  Inputs=++|
  Sum3 : Sum  Inputs=|-+
  Switch : Switch  Criteria=u2 > Threshold  Threshold=1e-5
  Q HX2 (W)7 : Outport
  Q HX2 (W)1 : Outport  Port=2
  Q HX2 (W)4 : Outport  Port=3
  Q HX2 (W)9 : Outport  Port=4
  Q HX2 (W)8 : Outport  Port=5
  Q HX2 (W)2 : Outport  Port=6
  Q HX2 (W)11 : Outport  Port=7
  wires:
  Constant/1 -> Switch/3
  Switch/1 -> Sum1/2
  Subsystem/6(Q HX2 (W)3) -> Product/2
  In1/1 -> Subsystem/1(In1), Sum1/1  "T1 in (K)"
  Sum1/1 -> Sum3/1, Q HX2 (W)7/1  "T1 out (K)"
  In6/1 -> Subsystem/6(In6)  "epsilon (0..1)"
  Subsystem/1(Q HX2 (W)8) -> Q HX2 (W)8/1  "NTU (1)"
  Subsystem/2(Q HX2 (W)9) -> Q HX2 (W)9/1  "UA (W/K)"
  In5/1 -> Subsystem/5(In5)  "dn/dt water (mol/sec)"
  In3/1 -> Subsystem/3(In3)  "P1 in = P1 out (bar)"
  Subsystem/4(Q HX2 (W)11) -> Q HX2 (W)11/1  "Cr (0..1)"
  In4/1 -> Subsystem/4(In4), Switch/2  "dn/dt 1 (mol/sec)"
  Subsystem/3(Q HX2 (W)10) -> Display/1  "q1→water max (W)"
  Subsystem/5(Q HX2 (W)4) -> Q HX2 (W)4/1, Product/1, Product1/1  "q1→water (W)"
  In7/1 -> Subsystem/7(In7), Sum2/1  "T water in (K)"
  Subsystem/7(Q HX2 (W)6) -> Product1/2
  Product1/1 -> Sum2/2  "Q * C2"
  Sum2/1 -> Q HX2 (W)1/1  "T water out (K)"
  Product/1 -> Switch/1  "Q * C1"
  Sum3/1 -> Q HX2 (W)2/1, Algebraic Constraint/1  "minimization residue"
  Algebraic Constraint/1 -> Sum3/2, Subsystem/2(In2)  "T1 out ** (K)"

== system thermochemical/Heat exchangers/Heat Exchanger, e-NTU method (epsilon input) One fluid or condensation//evaporation Loop 2: water ==
  In1 : Inport
  In7 : Inport  Port=2
  In5 : Inport  Port=3
  In6 : Inport  Port=4
  Display : Display
  NTU : Subsystem
  Product{,1..3} (4 alike) : Product
  Product4 : Product  Inputs=/*
  Sum : Sum  Inputs=+-
  Sum1 : Sum  Inputs=|++
  cp water (J/K·mol) : Constant  Value=cp_water_J_K_mol
  Q HX2 (W)1 : Outport
  Q HX2 (W)4 : Outport  Port=2
  Q HX2 (W)9 : Outport  Port=3
  Q HX2 (W)8 : Outport  Port=4
  wires:
  In7/1 -> Sum1/1, Sum/2  "T water in (K)"
  Product2/1 -> Product4/2, Q HX2 (W)4/1  "q1→water (W)"
  In5/1 -> Product3/2  "dn/dt water (mol/sec)"
  In6/1 -> NTU/1(In6), Product2/1  "epsilon (0..1)"
  In1/1 -> Sum/1  "T isotherm (K)"
  Sum1/1 -> Q HX2 (W)1/1  "T water out (K)"
  cp water (J/K·mol)/1 -> Product3/1  "cp2 avg (J/K·mol)"
  Product3/1 -> Product/1, Product4/1, Product1/2  "Cmin (W/K)"
  NTU/1(Q HX2 (W)8) -> Q HX2 (W)8/1, Product/2  "NTU (1)"
  Sum/1 -> Product1/1
  Product1/1 -> Display/1, Product2/2  "q1→2 max (W)"
  Product/1 -> Q HX2 (W)9/1  "UA (W/K)"
  Product4/1 -> Sum1/2

== system thermochemical/Heat exchangers/LMTD ==
  In4 : Inport
  In3 : Inport  Port=2
  In1 : Inport  Port=3
  In2 : Inport  Port=4
  Abs : Abs
  Abs1 : Abs
  Assertion (it gives error if input is zero) : Assertion  AssertionFailFcn=disp('Error. The values (T loop1,x=0 - T loop2,x=0) and (T loop1,x=L - T loop2,x=L) must have the same sign!')
  Display{1..6,9..10} (8 alike) : Display
  Divide6 : Product  Inputs=*/
  ERROR DETECTION : Subsystem
  Math Function : Math  Operator=log  SaturateOnIntegerOverflow=on
  Math Function1 : Math  Operator=log  SaturateOnIntegerOverflow=on
  Sum{1..4} (4 alike) : Sum  Inputs=+-
  Out2 : Outport
  wires:
  Sum2/1 -> ERROR DETECTION/1(In2), Abs/1, Display2/1
  Sum1/1 -> ERROR DETECTION/2(In1), Abs1/1, Display1/1
  Sum4/1 -> Display3/1, Divide6/2
  Math Function1/1 -> Display10/1, Sum4/2
  Math Function/1 -> Display9/1, Sum4/1
  Sum3/1 -> Display4/1, Divide6/1
  Divide6/1 -> Out2/1  "LMTD"
  In4/1 -> Sum2/1  "T loop1,x=0"
  In1/1 -> Sum1/1  "T loop1,x=L"
  In3/1 -> Sum2/2  "T loop2,x=0"
  In2/1 -> Sum1/2  "T loop2,x=L"
  Abs/1 -> Display6/1, Math Function/1, Sum3/1
  Abs1/1 -> Display5/1, Math Function1/1, Sum3/2
  ERROR DETECTION/1(Out2) -> Assertion (it gives error if input is zero)/1

== system thermochemical/Motors/DC motor + DC power supply + speed controller ==
  In1 : Inport
  In2 : Inport  Port=2
  In3 : Inport  Port=3
  "DC Power source, limited in its maximum instantaneous power" : Subsystem
  "DC motor, permanent magnet, one-way rotation" : thermochemical/Motors/DC motor, permanent magnet, one-way rotation  L=La_motor  R=Ra_motor  J=J_motor  b=b_motor  Km=Km_motor  w_init=w_init_motor
      settings: SourceProductName=@ Thermochemical
  PID Controller : simulink/Continuous/PID Controller  Controller=PID  TimeDomain=Continuous-time  SampleTime=-1  IntegratorMethod=Forward Euler  FilterMethod=Forward Euler  Form=Ideal  UseFilter=on  ControllerParametersSource=internal  P=PID_P  I=PID_I  D=PID_D  N=100  InitialConditionSource=internal  InitialConditionForIntegrator=0  InitialConditionForFilter=0  ExternalReset=none  LimitOutput=on  UpperSaturationLimit=V_max  LowerSaturationLimit=-V_max  LinearizeAsGain=off  AntiWindupMode=clamping  Kb=1  TrackingMode=off  Kt=1  PParamMin=[]  PParamMax=[]  IParamMin=[]  IParamMax=[]  DParamMin=[]  DParamMax=[]  NParamMin=[]  NParamMax=[]  KbParamMin=[]  KbParamMax=[]  KtParamMin=[]  KtParamMax=[]  POutMin=[]  POutMax=[]  IOutMin=[]  IOutMax=[]  DOutMin=[]  DOutMax=[]  NOutMin=[]  NOutMax=[]  KbOutMin=[]  KbOutMax=[]  KtOutMin=[]  KtOutMax=[]  IntegratorOutMin=[]  IntegratorOutMax=[]  FilterOutMin=[]  FilterOutMax=[]  SumOutMin=[]  SumOutMax=[]  SumI1OutMin=[]  SumI1OutMax=[]  SumI2OutMin=[]  SumI2OutMax=[]  SumI3OutMin=[]  SumI3OutMax=[]  SumDOutMin=[]  SumDOutMax=[]  SaturationOutMin=[]  SaturationOutMax=[]  IntegratorContinuousStateAttributes=''  IntegratorStateMustResolveToSignalObject=off  IntegratorRTWStateStorageClass=Auto  FilterContinuousStateAttributes=''  FilterStateMustResolveToSignalObject=off  FilterRTWStateStorageClass=Auto  DifferentiatorICPrevScaledInput=0  DifferentiatorOutMin=[]  DifferentiatorOutMax=[]  InitialConditionSetting=State (most efficient)  FilterDiffOutCoefMin=[]  FilterDiffOutCoefMax=[]  SumDenOutMin=[]  SumDenOutMax=[]  SumNumOutMin=[]  SumNumOutMax=[]  ReciprocalOutMin=[]  ReciprocalOutMax=[]  DivideOutMin=[]  DivideOutMax=[]  TunerSelectOption=Transfer Function Based (PID Tuner App)
  Sum : Sum  Inputs=|+-
  Terminator : Terminator
  Out1 : Outport
  Out2 : Outport  Port=2
  Out3 : Outport  Port=3
  Out4 : Outport  Port=4
  wires:
  In1/1 -> "DC Power source, limited in its maximum instantaneous power"/1(In3)  "Max power available (W)"
  In2/1 -> Sum/1  "ω ref (rad/sec)"
  In3/1 -> "DC motor, permanent magnet, one-way rotation"/1  "Torque load (N.m)"
  "DC motor, permanent magnet, one-way rotation"/4 -> Out1/1, Sum/2  "ω (rad/sec)"
  Sum/1 -> PID Controller/1  "error"
  PID Controller/1 -> "DC Power source, limited in its maximum instantaneous power"/2(In2)  "U ref (V)"
  "DC Power source, limited in its maximum instantaneous power"/1(Out1) -> "DC motor, permanent magnet, one-way rotation"/2  "U motor (V)"
  "DC motor, permanent magnet, one-way rotation"/5 -> "DC Power source, limited in its maximum instantaneous power"/3(In1)  "I motor (A)"
  "DC motor, permanent magnet, one-way rotation"/2 -> Out2/1  "Pow motor elec (W)"
  "DC Power source, limited in its maximum instantaneous power"/2(Out2) -> Terminator/1  "Clamp"
  "DC motor, permanent magnet, one-way rotation"/1 -> Out3/1  "Pow motor mech (W)"
  "DC motor, permanent magnet, one-way rotation"/3 -> Out4/1  "Pow load (W)"

== system thermochemical/Motors/DC motor, permanent magnet, one-way rotation ==
  note: The inferior saturation in the
      | integrator acts as a
      | reverse blocking system.
  In3 : Inport
  In1 : Inport  Port=2
  Divide1 : Product  Inputs=**
  Divide2 : Product  Inputs=**
  Divide3 : Product  Inputs=**
  Gain : Gain  Gain=1/L
  Gain1 : Gain  Gain=R
  Gain2 : Gain  Gain=Km
  Gain3 : Gain  Gain=Km
  Gain4 : Gain  Gain=1/J
  Gain5 : Gain  Gain=b
  Integrator Limited : Integrator  InitialCondition=w_init  LimitOutput=on  LowerSaturationLimit=0
  Integrator1 : Integrator
  Sum : Sum  Inputs=||+--
  Sum1 : Sum  Inputs=-+-
  Out4 : Outport
  Out3 : Outport  Port=2
  Out5 : Outport  Port=3
  Out1 : Outport  Port=4
  Out2 : Outport  Port=5
  wires:
  In1/1 -> Sum/1, Divide1/2  "U motor (V)"
  Integrator Limited/1 -> Gain3/1, Gain5/1, Divide3/2, Out1/1, Divide2/1  "ω (rad/sec)"
  In3/1 -> Divide3/1, Sum1/1  "Torque load (N.m)"
  Integrator1/1 -> Out2/1, Gain2/1, Divide1/1, Gain1/1  "I motor (A)"
  Sum/1 -> Gain/1
  Gain/1 -> Integrator1/1
  Gain1/1 -> Sum/3
  Gain2/1 -> Divide2/2, Sum1/2  "tao motor (N.m)"
  Sum1/1 -> Gain4/1
  Gain4/1 -> Integrator Limited/1
  Gain5/1 -> Sum1/3
  Gain3/1 -> Sum/2
  Divide1/1 -> Out3/1  "Pow elect (W)"
  Divide2/1 -> Out4/1  "Pow mech (W)"
  Divide3/1 -> Out5/1  "Pow load (W)"

== system thermochemical/Reactors/Reactor's internal energy equation ==
  In1 : Inport
  In3 : Inport  Port=2
  In2 : Inport  Port=3
  Binder : Subsystem
  Gas : Subsystem
  Salt : Subsystem
  Sum : Sum  Inputs=+++
  Out1 : Outport
  wires:
  In2/1 -> Gas/1(In2), Binder/1(In2), Salt/2(In2)  "Tr (K)"
  Sum/1 -> Out1/1  "U reactor (J)"
  Salt/1(Out1) -> Sum/1  "U salt (J)"
  In1/1 -> Salt/1(In1)  "X [0..1]"
  Binder/1(Out1) -> Sum/2  "U binder (J)"
  In3/1 -> Gas/2(In3)  "N_gas (void volume) (mol)"
  Gas/1(Out1) -> Sum/3  "U gas (J)"
